simulink model "sdl_manual_transmission_TEST"  (R2015a)
settings: Solver=ode23t  StartTime=0.0  StopTime=30  MaxStep=0.1  RelTol=1e-3
PreLoadFcn:
  | L=0;
undefined symbols (not defined in the file): sigbuilder_block
libraries: fl_lib x47, nesl_utility x12, sdl_lib x8
Description:
  | Vehicle With Manual Transmission
  | 
  | The vehicle simulated in this demo has a four-speed manual transmission,
  | a schematic for which is available in the Gearbox subsystem. The key
  | elements of the transmission are four synchronizers, denoted by S_1 to
  | S_4. By engaging or disengaging these synchronizers and associated dog
  | clutches, the transmission provides four ratios 3.581, 2.022, 1.384, and 1,
  | respectively. The synchronizers are modeled using the Cone Clutch block.
  | The model also provides an alternative abstracted representation of the
  | gearbox more suitable for hardware-in-the-loop simulation. To select this,
  | right-click the Gearbox subsystem, and select Block Choice -> Gearbox
  | (Abstracted).
  | 
  | 
  | Copyright 2008-2014 The MathWorks, Inc.
settings Model: CovSFcnEnable=off  Creator=MathWorks  LastModifiedBy=psanghvi
settings SolverCC: MaxConsecutiveZCs=10  MaxConsecutiveMinStep=5
settings DataIOCC: SignalLoggingSaveFormat=ModelDataLogs
settings OptimizationCC: ExpressionDepthLimit=2147483647
settings DebuggingCC: UnderspecifiedInitializationDetection=Classic  MergeDetectMultiDrivingBlocksExec=none  MaxConsecutiveZCsMsg=none  IgnoredZcDiagnostic=none  FcnCallInpInsideContextMsg=UseLocalSettings  StateNameClashWarn=warning
settings GRTTargetCC: CombineOutputUpdateFcns=off  GRTInterface=on

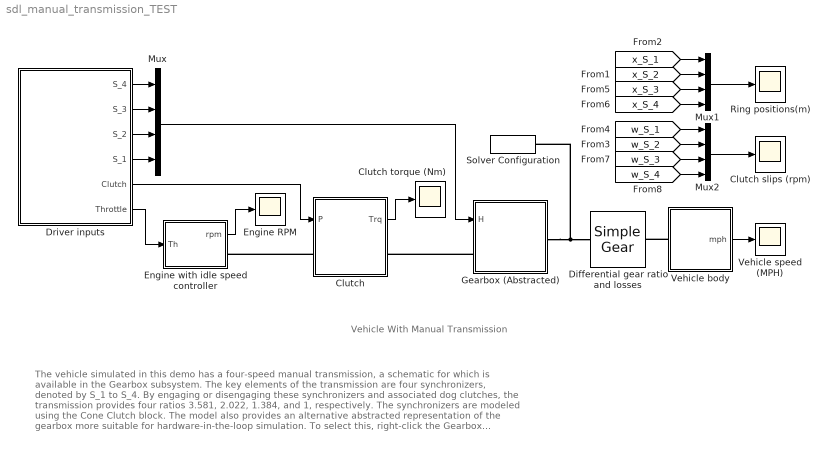
== system sdl_manual_transmission_TEST ==
  note: Vehicle With Manual Transmission
  note: The vehicle simulated in this demo has a four-speed manual transmission, a schematic for which is available in the Gearbox subsystem.
      | The key elements of the transmission are four synchronizers, denoted by S_1 to S_4. By engaging or disengaging these synchronizers and
      | associated dog clutches, the transmission provides four ratios 3.581, 2.022, 1.384, and 1, respectively. The synchronizers are modeled
      | using the Cone Clutch block. The model also provides an alternative abstracted representation of the gearbox more suitable for
      | hardware-in-the-loop simulation. To select this, right-click the Gearbox subsystem, and select Block Choice -> Gearbox (Abstracted).
  Clutch : Subsystem
  Clutch slips (rpm) : Scope
      settings: TimeRange=30  YMin=-2000  YMax=3000  SaveName=ScopeData8  MaxDataPoints=50000
  Clutch torque (Nm) : Scope
      settings: TimeRange=30  YMin=-50  YMax=300  SaveName=ScopeData4  MaxDataPoints=50000
  Differential gear ratio and losses : sdl_lib/Gears/Simple Gear  ratio=3.1  rotation_direction=1  friction_model=2  T_noload=0.1 N*m  T_nom=5 N*m  efficiency_nom=0.8  efficiency=0.86  mu_visc=[ L L ] N*m/(rad/s)  w_thr=0.01 rad/s  temperature_TLU=[ 280 300 320 ] K  load_TLU=[ 1 5 10 ] N*m  efficiency_TLU=[ 0.95 0.9 0.85 ]  efficiency_TLU2=[ 0.85 0.8 0.75; 0.95 0.9 0.85; 0.85 0.8 0.7 ]  thermal_mass=50 J/K  T_init=300 K
  Driver inputs : Subsystem  Tag=STV Subsys  LoadFcn=sigbuilder_block('load');  StartFcn=sigbuilder_block('start');  StopFcn=sigbuilder_block('stop');  ClipboardFcn=sigbuilder_block('clipboard');  mask(Sigbuilder block){}
      mask help: Sigbuilder GUI
      mask init:
      | if ~strcmp(get_param(bdroot(gcbh),'SimulationStatus'),'stopped') tuvar = sigbuilder_block('maskInit'); end
      settings: CopyFcn=sigbuilder_block('copy');  DeleteFcn=sigbuilder_block('delete');  ModelCloseFcn=sigbuilder_block('modelClose');  PreSaveFcn=sigbuilder_block('preSave');  PauseFcn=sigbuilder_block('pause')  ContinueFcn=sigbuilder_block('continue')  NameChangeFcn=sigbuilder_block('namechange');  OpenFcn=sigbuilder_block('open',[234.75 345 618.75 492 ]);  CloseFcn=sigbuilder_block('close');
      mask Display: plot(0,0,100,100,[10,10,40,40,10],[80,20,20,80,80],[40,10],[50,50], [40,27,10],[65,72,56],[40,25,25,10],[28,28,43,43]);
  Engine RPM : Scope
      settings: TimeRange=30  YMin=0  YMax=6000  SaveName=ScopeData6  MaxDataPoints=50000
  Engine with idle speed controller : Subsystem
  Gearbox (Abstracted) : Subsystem
  Mux : Mux
  Mux1 : Mux
  Mux2 : Mux
  Ring positions(m) : Scope
      settings: TimeRange=30  YMin=-0.005  YMax=0.015  SaveName=ScopeData7  MaxDataPoints=50000
  Solver Configuration : nesl_utility/Solver Configuration  PhysicalDomain=network_engine_domain  SubClassName=solver  LeftPortType=input  RightPortType=generic  Accelerate=off  Tones=[]  Harmonics=[]  SimulateNoise=off  Profile=off  UseLocalSampling=off  EnableSwitchedLinearOptims=on  FrequencyDomain=off  UseCCode=off  RelTol=0.001  AbsTol=1e-06  MinStep=1e-09  ToWorkspace=off  RevertToSquareIcSolve=off  NumHomotopyIterations=100  DoDC=off  ResidualTolerance=1e-9  UseLocalSolver=off  LocalSolverChoice=NE_BACKWARD_EULER_ADVANCER  LocalSolverSampleTime=.001  DoFixedCost=off  MaxNonlinIter=10  MaxModeIter=2  LinearAlgebra=Sparse  DelaysMemoryBudget=1024  AutomaticFiltering=on  FilteringTimeConstant=0.001
  Vehicle speed (MPH) : Scope
      settings: TimeRange=30  YMin=-20  YMax=80  SaveName=ScopeData5  MaxDataPoints=50000
  Vehicle body : Subsystem
  wires:
  Driver inputs/2(S_3) -> Mux/2
  Driver inputs/1(S_4) -> Mux/1
  Driver inputs/3(S_2) -> Mux/3
  Driver inputs/4(S_1) -> Mux/4
  Driver inputs/6(Throttle) -> Engine with idle speed controller/1(Th)
  Mux/1 -> Gearbox (Abstracted)/1(H)
  Driver inputs/5(Clutch) -> Clutch/1(P)
  Vehicle body/1(mph) -> Vehicle speed (MPH)/1
  Engine with idle speed controller/1(rpm) -> Engine RPM/1
  Clutch/1(Trq) -> Clutch torque (Nm)/1
  [x_S_1] -> Mux1/1
  [x_S_2] -> Mux1/2
  Mux1/1 -> Ring positions(m)/1
  Mux2/1 -> Clutch slips (rpm)/1
  [x_S_3] -> Mux1/3
  [x_S_4] -> Mux1/4
  [w_S_1] -> Mux2/1
  [w_S_2] -> Mux2/2
  [w_S_3] -> Mux2/3
  [w_S_4] -> Mux2/4
  connections:
  Clutch/LConn1 -- Engine with idle speed controller/RConn1
  Vehicle body/LConn1 -- Differential gear ratio and losses/RConn1
  Gearbox (Abstracted)/LConn1 -- Clutch/RConn1
  Gearbox (Abstracted)/RConn1 -- Differential gear ratio and losses/LConn1 -- Solver Configuration/RConn1

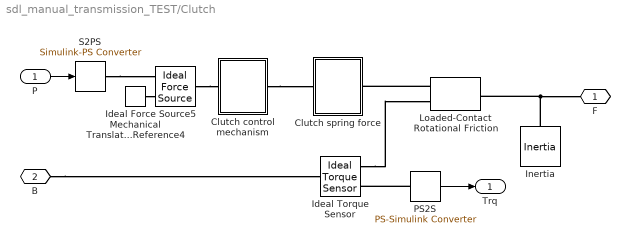
== system sdl_manual_transmission_TEST/Clutch ==
  P : Inport
  Clutch control mechanism : Subsystem
  Clutch spring force : Subsystem
  Ideal Torque Sensor : fl_lib/Mechanical/Mechanical Sensors/Ideal Torque Sensor
  Ideal Force Source5 : fl_lib/Mechanical/Mechanical Sources/Ideal Force Source
  Inertia : fl_lib/Mechanical/Rotational Elements/Inertia  inertia=0.005 kg*m^2  w_specify=on  w_priority=High  w=0 rad/s  t_specify=off  t_priority=High  t=0 N*m
  Loaded-Contact Rotational Friction : sdl_lib/Brakes & Detents/Rotational/Loaded-Contact Rotational Friction  geometry_model=1  r_eff=300 mm  d_o=150 mm  d_i=100 mm  friction_model=1  mu_coulomb=0.46  mu_w_vector=[ 0 0.1 0.2 0.3 0.4 0.5 1 2 5 10 100 1000 ] rad/s  mu_coulomb_vector=[ 0.29 0.28 0.26 0.22 0.21 0.2 0.2 0.19 0.19 0.19 0.19 0.19 ]  mu_interp_method=1  mu_extrap_method=1  mu_static=0.5  w_tol=0.001 rad/s  force_min=10 N  mu_visc=0 N*m/(rad/s)  initial_state_locked=0
  Mechanical Translational Reference4 : fl_lib/Mechanical/Translational Elements/Mechanical Translational Reference
  PS2S : nesl_utility/PS-Simulink Converter  PhysicalDomain=network_engine_domain  SubClassName=ps_output  LeftPortType=input  RightPortType=output  PseudoPeriodic=off  Frequencies=[]  Unit=1  AffineConversion=off
  S2PS : nesl_utility/Simulink-PS Converter  PhysicalDomain=network_engine_domain  SubClassName=ps_input  LeftPortType=input  RightPortType=output  PseudoPeriodic=off  Frequencies=[]  NoiseDistribution=none  NoiseParameters=[]  Unit=1  AffineConversion=off  InputFiltering=off  SimscapeFilterOrder=1  InputFilterTimeConstant=.001  UdotUserProvided=0
  F : PMIOPort  Port=1  Side=Right
  B : PMIOPort  Port=2  Side=Left
  Trq : Outport
  wires:
  P/1 -> S2PS/1
  PS2S/1 -> Trq/1
  connections:
  Mechanical Translational Reference4/LConn1 -- Ideal Force Source5/RConn2
  S2PS/RConn1 -- Ideal Force Source5/RConn1
  Ideal Force Source5/LConn1 -- Clutch control mechanism/LConn1
  Inertia/LConn1 -- Loaded-Contact Rotational Friction/RConn1 -- F/RConn1
  PS2S/LConn1 -- Ideal Torque Sensor/RConn2
  Clutch control mechanism/RConn1 -- Clutch spring force/LConn1
  Loaded-Contact Rotational Friction/LConn1 -- Clutch spring force/RConn1
  Ideal Torque Sensor/RConn1 -- Loaded-Contact Rotational Friction/LConn2
  B/RConn1 -- Ideal Torque Sensor/LConn1

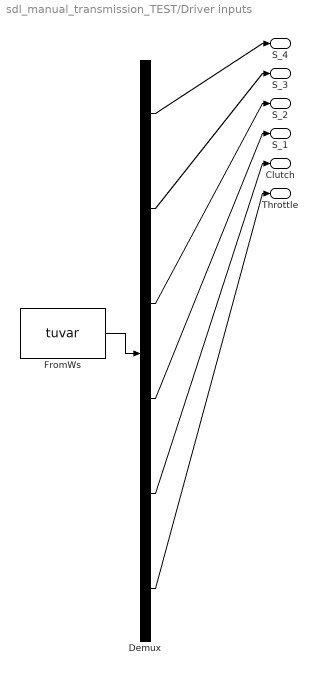
== system sdl_manual_transmission_TEST/Driver inputs ==
  Demux : Demux  Tag=STV Demux  Outputs=6
  FromWs : FromWorkspace  Tag=STV FromWs  VariableName=tuvar  SampleTime=0
      SigBuilderData=|
      | common.afterFinalStr = 'Extrapolate'
      | common.sampleTime = 0
      | dataSet.timeRange = [0 30]
      | dataSet.name = 'Group 1'
      | sbobj.Groups.Name = 'Group 1'
      | sbobj.Groups.Signals(1).Name = 'S_4'
      | sbobj.Groups.Signals(1).XData = [0 23.3 23.5 24 24.3 30]
      | sbobj.Groups.Signals(1).YData = [0 0 250 250 0 0]
      | sbobj.Groups.Signals(2).Name = 'S_3'
      | sbobj.Groups.Signals(2).XData = [0 16.1 16.3 16.9 17.2 22.8 23 23.6 23.7 30]
      | sbobj.Groups.Signals(2).YData = [0 0 250 250 0 0 -250 -250 0 0]
      | sbobj.Groups.Signals(3).Name = 'S_2'
      | sbobj.Groups.Signals(3).XData = [0 8.8 9 9.5 9.75 15.8 16.05 16.6 16.8 30]
      | sbobj.Groups.Signals(3).YData = [0 0 250 250 0 0 -250 -250 0 0]
      | sbobj.Groups.Signals(4).Name = 'S_1'
      | sbobj.Groups.Signals(4).XData = [0 1.7 1.85 3.15 3.35 8.35 8.5 9.3 9.4 30]
      | sbobj.Groups.Signals(4).YData = [0 0 250 250 0 0 -250 -250 0 0]
      | sbobj.Groups.Signals(5).Name = 'Clutch'
      | sbobj.Groups.Signals(5).XData = [0 0.95 1.45 3.5 4 8.15 8.35 10 10.4 15.4 15.8 17.2 17.7 22.5 22.8 24.3 24.6 30]
      | sbobj.Groups.Signals(5).YData = [0 0 120 120 -0.05 0 120 120 0 0 120 120 0 0 120 120 0 0]
      | sbobj.Groups.Signals(6).Name = 'Throttle'
      | sbobj.Groups.Signals(6).XData = [0 3.2 4 7.45 7.6 10.25 10.4 15 15.2 17.6 17.8 22.35 22.6 24.6 24.8 30]
      | sbobj.Groups.Signals(6).YData = [0 0 0.95 0.95 0 0 0.96 0.943121387283 0 0 1 1 0 0 1 1]
      | sbobj.Groups.TimeRange = [0 30]
  S_4 : Outport  Tag=STV Outport
  S_3 : Outport  Tag=STV Outport  Port=2
  S_2 : Outport  Tag=STV Outport  Port=3
  S_1 : Outport  Tag=STV Outport  Port=4
  Clutch : Outport  Tag=STV Outport  Port=5
  Throttle : Outport  Tag=STV Outport  Port=6
  wires:
  Demux/6 -> Throttle/1
  Demux/5 -> Clutch/1
  Demux/4 -> S_1/1
  Demux/3 -> S_2/1
  Demux/2 -> S_3/1
  Demux/1 -> S_4/1
  FromWs/1 -> Demux/1

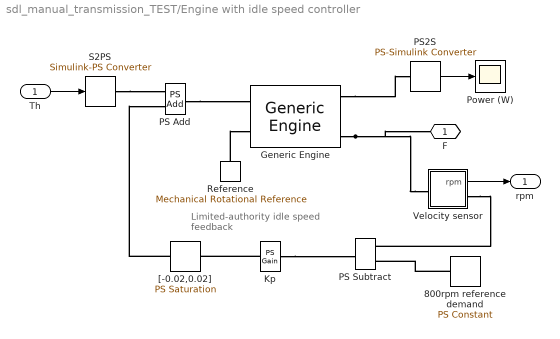
== system sdl_manual_transmission_TEST/Engine with idle speed controller ==
  note: Limited-authority
      | idle speed feedback
  Th : Inport
  800rpm reference demand : fl_lib/Physical Signals/Sources/PS Constant  constant=800*2*pi/60
  Generic Engine : sdl_lib/Engines/Generic Engine  model_parameterization=1  engine_type=1  P_max=100e3 W  w_P_max=4.5e+3 rpm  w_max=6e+3 rpm  w_min=200 rpm  w_tab=[ 500 1000 2e+3 3e+3 4e+3 5e+3 6e+3 7e+3 ] rpm  trq_tab=[ 380 380 380 380 350 280 200 80 ] N*m  pwr_tab=[ 2e+4 4e+4 7.8e+4 1.2e+5 1.45e+5 1.48e+5 1.25e+5 6e+4 ] W  interp_method=1  model_inertia=1  inertia=0.08 kg*m^2  initial_velocity=800 rpm  model_time_constant=1  time_constant=0.2 s  T0=0  w_thr=20 rpm  idle_speed=0  idle_speed_reference=1000 rpm  tau_controller=1 s  idle_w_thr=1 rpm  fc_model=1  fc_per_rev=25 mg/rev  displaced_volume=400 cm^3  rev_per_cycle=2  fc_w_tab=[ 1000 2e+3 3e+3 4e+3 5e+3 6e+3 ] rpm  fc_trq_tab=[ 0 80 160 200 240 320 360 400 ] N*m  fc_tab=[ 0.5 0.9 1.4 1.6 1.9 2.7 3.4 4.4; 1 1.7 2.7 3.1 3.6 5 6 7.4; 1.4 2.7 4 4.8 5.6 7.5 8.5 10.5; 2 3.6 5.8 6.7 8 10.4 11.7 13.3; 2.5 4.8 7.9 9.4 10.8 14 16.2 18.6; 3.1 6 10.3 11.9 13.8 18.4 22 26.5 ] g/s  bmep_tab=[ 0 250 500 625 750 1000 1.15e+3 1.25e+3 ] kPa  bsfc_tab=[ 410 380 300 280 270 290 320 380; 410 370 290 270 260 270 285 320; 415 380 290 275 265 270 270 300; 420 390 310 290 285 280 280 285; 430 410 340 320 310 300 310 320; 450 430 370 340 330 330 350 380 ] g/hr/kW  fc_interp_method=1
  Kp : fl_lib/Physical Signals/Functions/PS Gain  gain=0.005
  PS Add : fl_lib/Physical Signals/Functions/PS Add
  PS Subtract : fl_lib/Physical Signals/Functions/PS Subtract
  PS2S : nesl_utility/PS-Simulink Converter  PhysicalDomain=network_engine_domain  SubClassName=ps_output  LeftPortType=input  RightPortType=output  PseudoPeriodic=off  Frequencies=[]  Unit=1  AffineConversion=off
  Power (W) : Scope
      settings: TimeRange=15  YMin=-50000  YMax=150000  SaveName=ScopeData2
  Reference : fl_lib/Mechanical/Rotational Elements/Mechanical Rotational Reference
  S2PS : nesl_utility/Simulink-PS Converter  PhysicalDomain=network_engine_domain  SubClassName=ps_input  LeftPortType=input  RightPortType=output  PseudoPeriodic=off  Frequencies=[]  NoiseDistribution=none  NoiseParameters=[]  Unit=1  AffineConversion=off  InputFiltering=off  SimscapeFilterOrder=1  InputFilterTimeConstant=.001  UdotUserProvided=0
  Velocity sensor : Subsystem
  "[-0.02,0.02]" : fl_lib/Physical Signals/Nonlinear Operators/PS Saturation  upper_limit=0.02  lower_limit=-0.02
  F : PMIOPort  Port=1  Side=Right
  rpm : Outport
  wires:
  Velocity sensor/1(rpm) -> rpm/1
  PS2S/1 -> Power (W)/1
  Th/1 -> S2PS/1
  connections:
  Generic Engine/RConn1 -- PS2S/LConn1
  Reference/LConn1 -- Generic Engine/LConn2
  PS Add/RConn1 -- Generic Engine/LConn1
  S2PS/RConn1 -- PS Add/LConn1
  Velocity sensor/RConn1 -- PS Subtract/LConn2
  800rpm reference demand/RConn1 -- PS Subtract/LConn1
  Kp/LConn1 -- PS Subtract/RConn1
  "[-0.02,0.02]"/RConn1 -- PS Add/LConn2
  Kp/RConn1 -- "[-0.02,0.02]"/LConn1
  Velocity sensor/LConn1 -- Generic Engine/RConn3 -- F/RConn1

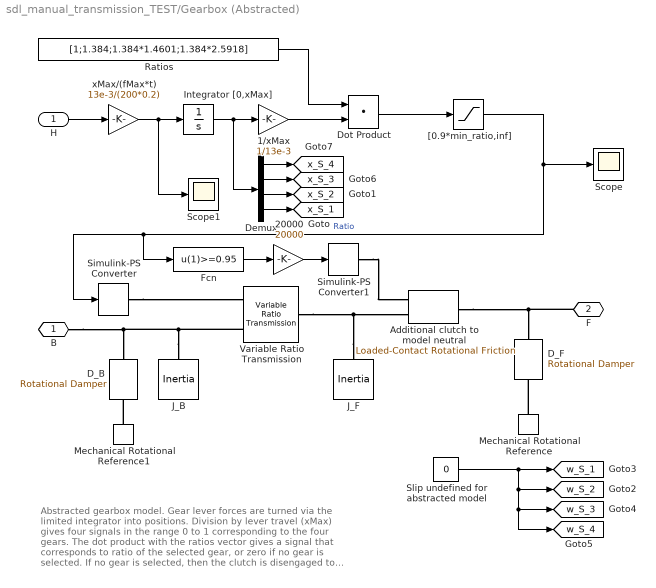
== system sdl_manual_transmission_TEST/Gearbox (Abstracted) ==
  note: Abstracted gearbox model. Gear lever forces are turned
      | via the limited integrator into positions. Division
      | by lever travel (xMax) gives four signals in the range
      | 0 to 1 corresponding to the four gears. The dot
      | product with the ratios vector gives a signal that
      | corresponds to ratio of the selected gear, or zero if
      | no gear is selected. If no gear is selected, then the
      | clutch is disengaged to represent neutral.
  H : Inport
  1/xMax : Gain  Gain=1/13e-3  SaturateOnIntegerOverflow=on  OutDataTypeStr=Inherit: Same as input  ParamDataTypeStr=Inherit: Same as input
  20000 : Gain  Gain=20000  SaturateOnIntegerOverflow=on  OutDataTypeStr=Inherit: Same as input  ParamDataTypeStr=Inherit: Same as input
  Additional clutch to model neutral : sdl_lib/Brakes & Detents/Rotational/Loaded-Contact Rotational Friction  geometry_model=1  r_eff=300 mm  d_o=150 mm  d_i=100 mm  friction_model=1  mu_coulomb=0.46  mu_w_vector=[ 0 0.1 0.2 0.3 0.4 0.5 1 2 5 10 100 1000 ] rad/s  mu_coulomb_vector=[ 0.29 0.28 0.26 0.22 0.21 0.2 0.2 0.19 0.19 0.19 0.19 0.19 ]  mu_interp_method=1  mu_extrap_method=1  mu_static=0.5  w_tol=0.001 rad/s  force_min=100 N  mu_visc=0 N*m/(rad/s)  initial_state_locked=0
  D_B : fl_lib/Mechanical/Rotational Elements/Rotational Damper  D=0.01 N*m/(rad/s)  w_specify=off  w_priority=High  w=0 rad/s  t_specify=off  t_priority=High  t=0 N*m
  D_F : fl_lib/Mechanical/Rotational Elements/Rotational Damper  D=0.01 N*m/(rad/s)  w_specify=off  w_priority=High  w=0 rad/s  t_specify=off  t_priority=High  t=0 N*m
  Demux : Demux
  Dot Product : DotProduct  OutDataTypeStr=Inherit: Inherit via internal rule
  Fcn : Fcn  Expr=u(1)>=0.95
  Integrator [0,xMax] : Integrator  LimitOutput=on  UpperSaturationLimit=13e-3  LowerSaturationLimit=0
  J_B : fl_lib/Mechanical/Rotational Elements/Inertia  inertia=0.026 kg*m^2  w_specify=on  w_priority=High  w=0 rad/s  t_specify=off  t_priority=High  t=0 N*m
  J_F : fl_lib/Mechanical/Rotational Elements/Inertia  inertia=0.034 kg*m^2  w_specify=on  w_priority=High  w=0 rad/s  t_specify=off  t_priority=High  t=0 N*m
  Mechanical Rotational Reference : fl_lib/Mechanical/Rotational Elements/Mechanical Rotational Reference
  Mechanical Rotational Reference1 : fl_lib/Mechanical/Rotational Elements/Mechanical Rotational Reference
  Ratios : Constant  Value=[1;1.384;1.384*1.4601;1.384*2.5918]  VectorParams1D=off
  Scope : Scope
  Scope1 : Scope
      settings: SaveName=ScopeData9
  Simulink-PS Converter : nesl_utility/Simulink-PS Converter  PhysicalDomain=network_engine_domain  SubClassName=ps_input  LeftPortType=input  RightPortType=output  PseudoPeriodic=off  Frequencies=[]  NoiseDistribution=none  NoiseParameters=[]  Unit=1  AffineConversion=off  InputFiltering=off  SimscapeFilterOrder=1  InputFilterTimeConstant=.001  UdotUserProvided=0
  Simulink-PS Converter1 : nesl_utility/Simulink-PS Converter  PhysicalDomain=network_engine_domain  SubClassName=ps_input  LeftPortType=input  RightPortType=output  PseudoPeriodic=off  Frequencies=[]  NoiseDistribution=none  NoiseParameters=[]  Unit=1  AffineConversion=off  InputFiltering=off  SimscapeFilterOrder=1  InputFilterTimeConstant=.001  UdotUserProvided=0
  Slip undefined for abstracted model : Constant  Value=0
  Variable Ratio Transmission : sdl_lib/Couplings & Drives/Variable Ratio Transmission  rotation_direction=1  kp=1e+5 N*m/rad  kv=10 N*m/(rad/s)  initial_torque=0 N*m  losses_model=1  efficiency=0.85  mu_visc=[ 0 0 ] N*m/(rad/s)  w_thr=0.01 rad/s
  "[0.9*min_ratio,inf]" : Saturate  UpperLimit=inf  LowerLimit=0.9
  xMax/(fMax*t) : Gain  Gain=13e-3/(200*0.2)  SaturateOnIntegerOverflow=on  OutDataTypeStr=Inherit: Same as input  ParamDataTypeStr=Inherit: Same as input
  B : PMIOPort  Port=1  Side=Left
  F : PMIOPort  Port=2  Side=Right
  tag scope: w_S_1=global, w_S_2=global, w_S_3=global, w_S_4=global, x_S_1=global, x_S_2=global, x_S_3=global, x_S_4=global
  wires:
  Dot Product/1 -> "[0.9*min_ratio,inf]"/1
  Ratios/1 -> Dot Product/1
  1/xMax/1 -> Dot Product/2
  Integrator [0,xMax]/1 -> 1/xMax/1, Demux/1
  xMax/(fMax*t)/1 -> Integrator [0,xMax]/1, Scope1/1
  H/1 -> xMax/(fMax*t)/1
  Demux/4 -> [x_S_1]
  Demux/3 -> [x_S_2]
  Demux/1 -> [x_S_4]
  Demux/2 -> [x_S_3]
  "[0.9*min_ratio,inf]"/1 -> Simulink-PS Converter/1, Fcn/1, Scope/1  "Ratio"
  Fcn/1 -> 20000/1
  20000/1 -> Simulink-PS Converter1/1
  Slip undefined for abstracted model/1 -> [w_S_4], [w_S_3], [w_S_2], [w_S_1]
  connections:
  F/RConn1 -- D_F/LConn1 -- Additional clutch to model neutral/RConn1
  Mechanical Rotational Reference1/LConn1 -- D_B/RConn1
  Mechanical Rotational Reference/LConn1 -- D_F/RConn1
  J_B/LConn1 -- D_B/LConn1 -- B/RConn1 -- Variable Ratio Transmission/LConn2
  Simulink-PS Converter/RConn1 -- Variable Ratio Transmission/LConn1
  J_F/LConn1 -- Additional clutch to model neutral/LConn2 -- Variable Ratio Transmission/RConn1
  Simulink-PS Converter1/RConn1 -- Additional clutch to model neutral/LConn1

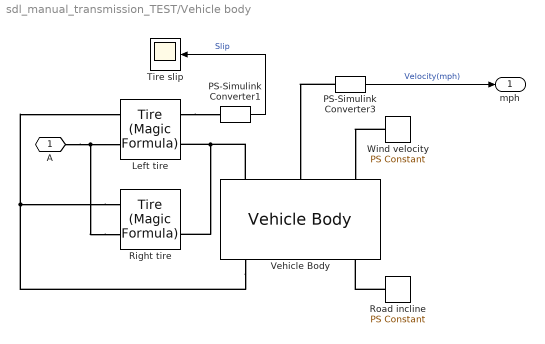
== system sdl_manual_transmission_TEST/Vehicle body ==
  Left tire : sdl_lib/Tires & Vehicles/Tire (Magic Formula)  parameterization=3  F_z1=3000 N  F_x1=3500 N  kappa1=10  B_m=10  C_m=1.9  D_m=1  E_m=0.97  fz0=4e+3 N  p_Cx=1.685  p_Dx=[ 1.21 -0.037 ]  p_Ex=[ 0.344 0.095 -0.02 0 ]  p_Kx=[ 21.51 -0.163 0.245 ]  p_Hx=[ -0.002 0.002 ]  p_Vx=[ 0 0 ]  v_tr_thr=0.1 m/s  r_e=0.4 m  model_compliance=0  stiffness=1e+6 N/m  damping=1000 N/(m/s)  model_inertia=1  inertia=0.8 kg*m^2  initial_velocity=0 rpm  model_resistance=0  resistance_model=1  coeff=0.015  p_tire=250e3 Pa  alpha=-0.003  beta=0.97  coeff_a=84e-4  coeff_b=6.2e-4 s/m  coeff_c=1.6e-4 s^2/m^2  v_thr=1e-3 m/s
  PS-Simulink Converter1 : nesl_utility/PS-Simulink Converter  PhysicalDomain=network_engine_domain  SubClassName=ps_output  LeftPortType=input  RightPortType=output  PseudoPeriodic=off  Frequencies=[]  Unit=1  AffineConversion=off
  PS-Simulink Converter3 : nesl_utility/PS-Simulink Converter  PhysicalDomain=network_engine_domain  SubClassName=ps_output  LeftPortType=input  RightPortType=output  PseudoPeriodic=off  Frequencies=[]  Unit=mph  AffineConversion=off
  Right tire : sdl_lib/Tires & Vehicles/Tire (Magic Formula)  parameterization=3  F_z1=3000 N  F_x1=3500 N  kappa1=10  B_m=10  C_m=1.9  D_m=1  E_m=0.97  fz0=4e+3 N  p_Cx=1.685  p_Dx=[ 1.21 -0.037 ]  p_Ex=[ 0.344 0.095 -0.02 0 ]  p_Kx=[ 21.51 -0.163 0.245 ]  p_Hx=[ -0.002 0.002 ]  p_Vx=[ 0 0 ]  v_tr_thr=0.1 m/s  r_e=0.4 m  model_compliance=0  stiffness=1e+6 N/m  damping=1000 N/(m/s)  model_inertia=1  inertia=0.8 kg*m^2  initial_velocity=0 rpm  model_resistance=0  resistance_model=1  coeff=0.015  p_tire=250e3 Pa  alpha=-0.003  beta=0.97  coeff_a=84e-4  coeff_b=6.2e-4 s/m  coeff_c=1.6e-4 s^2/m^2  v_thr=1e-3 m/s
  Road incline : fl_lib/Physical Signals/Sources/PS Constant  constant=0
  Tire slip : Scope
      settings: YMin=0  YMax=0.1  SaveName=ScopeData3  MaxDataPoints=500000  SampleTime=0.1
  Vehicle Body : sdl_lib/Tires & Vehicles/Vehicle Body  mass=1200 kg  n_w=2  x_f=1.4 m  x_r=1.6 m  y_c=0.5 m  area=3 m^2  Cd=0.4  v0=0 m/s  g=9.81 m/s^2  rho=1.18 kg/m^3
  Wind velocity : fl_lib/Physical Signals/Sources/PS Constant  constant=5
  A : PMIOPort  Port=1  Side=Left
  mph : Outport
  wires:
  PS-Simulink Converter3/1 -> mph/1  "Velocity(mph)"
  PS-Simulink Converter1/1 -> Tire slip/1  "Slip"
  connections:
  Right tire/RConn2 -- Left tire/RConn2 -- Vehicle Body/LConn1
  Right tire/LConn1 -- Left tire/LConn1 -- Vehicle Body/RConn1
  Right tire/LConn2 -- Left tire/LConn2 -- A/RConn1
  PS-Simulink Converter3/LConn1 -- Vehicle Body/LConn2
  Wind velocity/RConn1 -- Vehicle Body/LConn3
  Road incline/RConn1 -- Vehicle Body/RConn3
  Left tire/RConn1 -- PS-Simulink Converter1/LConn1

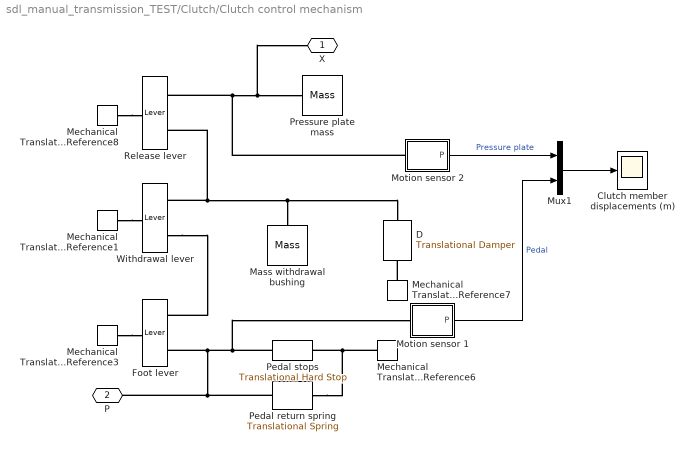
== system sdl_manual_transmission_TEST/Clutch/Clutch control mechanism ==
  Clutch member displacements (m) : Scope
      settings: TimeRange=15  YMin=-0.05  YMax=0.2  MaxDataPoints=50000
  D : fl_lib/Mechanical/Translational Elements/Translational Damper  D=100 N/(m/s)  v_specify=off  v_priority=High  v=0 m/s  f_specify=off  f_priority=High  f=0 N
  Foot lever : fl_lib/Mechanical/Mechanisms/Lever  arm_AC=76 mm  arm_BC=148 mm  f_A_specify=off  f_A_priority=High  f_A=0 N  f_B_specify=off  f_B_priority=High  f_B=0 N  f_C_specify=off  f_C_priority=High  f_C=0 N
  Mass withdrawal bushing : fl_lib/Mechanical/Translational Elements/Mass  mass=0.6 kg  v_specify=on  v_priority=High  v=0 m/s  f_specify=off  f_priority=High  f=0 N
  Mechanical Translational Reference{1,3,6..8} (5 alike) : fl_lib/Mechanical/Translational Elements/Mechanical Translational Reference
  Motion sensor 1 : Subsystem
  Motion sensor 2 : Subsystem
  Mux1 : Mux  Inputs=2
  Pedal return spring : fl_lib/Mechanical/Translational Elements/Translational Spring  spr_rate=120 N/m  v_specify=off  v_priority=High  v=0 m/s  f_specify=off  f_priority=High  f=0 N  x_specify=on  x_priority=High  x=1.5 cm
  Pedal stops : fl_lib/Mechanical/Translational Elements/Translational Hard Stop  upper_bnd=168 mm  lower_bnd=0 mm  stiff_up=1e6 N/m  stiff_low=1e6 N/m  D_up=150 N/(m/s)  D_low=150 N/(m/s)  v_specify=off  v_priority=High  v=0 m/s  f_specify=off  f_priority=High  f=0 N  x_specify=on  x_priority=High  x=0 m
  Pressure plate mass : fl_lib/Mechanical/Translational Elements/Mass  mass=4.2 kg  v_specify=on  v_priority=High  v=0 m/s  f_specify=off  f_priority=High  f=0 N
  Release lever : fl_lib/Mechanical/Mechanisms/Lever  arm_AC=7.2 mm  arm_BC=38 mm  f_A_specify=off  f_A_priority=High  f_A=0 N  f_B_specify=off  f_B_priority=High  f_B=0 N  f_C_specify=off  f_C_priority=High  f_C=0 N
  Withdrawal lever : fl_lib/Mechanical/Mechanisms/Lever  arm_AC=42 mm  arm_BC=128 mm  f_A_specify=off  f_A_priority=High  f_A=0 N  f_B_specify=off  f_B_priority=High  f_B=0 N  f_C_specify=off  f_C_priority=High  f_C=0 N
  X : PMIOPort  Port=1  Side=Right
  P : PMIOPort  Port=2  Side=Left
  wires:
  Motion sensor 2/1(P) -> Mux1/1  "Pressure plate"
  Motion sensor 1/1(P) -> Mux1/2  "Pedal"
  Mux1/1 -> Clutch member displacements (m)/1
  connections:
  Mechanical Translational Reference3/LConn1 -- Foot lever/RConn1
  Mechanical Translational Reference6/LConn1 -- Pedal stops/RConn1 -- Pedal return spring/RConn1
  Mechanical Translational Reference7/LConn1 -- D/RConn1
  Mechanical Translational Reference8/LConn1 -- Release lever/RConn1
  Withdrawal lever/LConn2 -- Foot lever/LConn1
  Mechanical Translational Reference1/LConn1 -- Withdrawal lever/RConn1
  Withdrawal lever/LConn1 -- Release lever/LConn2 -- Mass withdrawal bushing/LConn1 -- D/LConn1
  Motion sensor 2/LConn1 -- Release lever/LConn1 -- X/RConn1 -- Pressure plate mass/LConn1
  Pedal stops/LConn1 -- Foot lever/LConn2 -- Pedal return spring/LConn1 -- P/RConn1 -- Motion sensor 1/LConn1

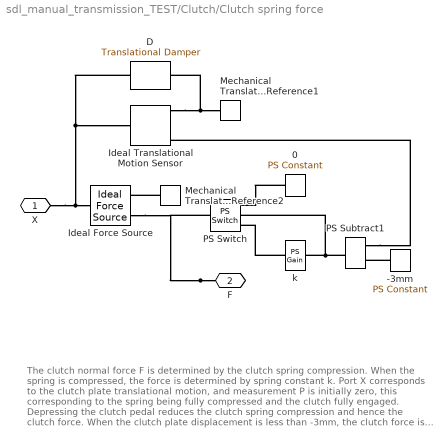
== system sdl_manual_transmission_TEST/Clutch/Clutch spring force ==
  note: The clutch normal force F is determined by the clutch spring compression.
      | When the spring is compressed, the force is determined by spring constant
      | k. Port X corresponds to the clutch plate translational motion, and
      | measurement P is initially zero, this corresponding to the spring being
      | fully compressed and the clutch fully engaged. Depressing the clutch pedal
      | reduces the clutch spring compression and hence the clutch force. When the
      | clutch plate displacement is less than -3mm, the clutch force is zero, and
      | hence it is fully disengaged.
  -3mm : fl_lib/Physical Signals/Sources/PS Constant  constant=-3e-3
  0 : fl_lib/Physical Signals/Sources/PS Constant  constant=0
  D : fl_lib/Mechanical/Translational Elements/Translational Damper  D=100 N/(m/s)  v_specify=off  v_priority=High  v=0 m/s  f_specify=off  f_priority=High  f=0 N
  Ideal Force Source : fl_lib/Mechanical/Mechanical Sources/Ideal Force Source
  Ideal Translational Motion Sensor : fl_lib/Mechanical/Mechanical Sensors/Ideal Translational Motion Sensor  offset=0 m
  Mechanical Translational Reference1 : fl_lib/Mechanical/Translational Elements/Mechanical Translational Reference
  Mechanical Translational Reference2 : fl_lib/Mechanical/Translational Elements/Mechanical Translational Reference
  PS Subtract1 : fl_lib/Physical Signals/Functions/PS Subtract
  PS Switch : fl_lib/Physical Signals/Nonlinear Operators/PS Switch  Threshold=0
  k : fl_lib/Physical Signals/Functions/PS Gain  gain=2000/3e-3
  X : PMIOPort  Port=1  Side=Left
  F : PMIOPort  Port=2  Side=Right
  connections:
  Ideal Translational Motion Sensor/RConn1 -- Mechanical Translational Reference1/LConn1 -- D/RConn1
  PS Subtract1/LConn1 -- Ideal Translational Motion Sensor/RConn3
  D/LConn1 -- X/RConn1 -- Ideal Force Source/LConn1 -- Ideal Translational Motion Sensor/LConn1
  F/RConn1 -- Ideal Force Source/RConn1 -- PS Switch/RConn1
  Mechanical Translational Reference2/LConn1 -- Ideal Force Source/RConn2
  PS Subtract1/RConn1 -- k/LConn1 -- PS Switch/LConn2
  k/RConn1 -- PS Switch/LConn1
  0/RConn1 -- PS Switch/LConn3
  -3mm/RConn1 -- PS Subtract1/LConn2

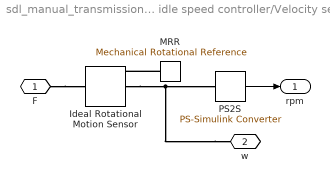
== system sdl_manual_transmission_TEST/Engine with idle speed controller/Velocity sensor ==
  Ideal Rotational Motion Sensor : fl_lib/Mechanical/Mechanical Sensors/Ideal Rotational Motion Sensor  offset=0 rad
  MRR : fl_lib/Mechanical/Rotational Elements/Mechanical Rotational Reference
  PS2S : nesl_utility/PS-Simulink Converter  PhysicalDomain=network_engine_domain  SubClassName=ps_output  LeftPortType=input  RightPortType=output  PseudoPeriodic=off  Frequencies=[]  Unit=rpm  AffineConversion=off
  F : PMIOPort  Port=1  Side=Left
  w : PMIOPort  Port=2  Side=Right
  rpm : Outport
  wires:
  PS2S/1 -> rpm/1
  connections:
  F/RConn1 -- Ideal Rotational Motion Sensor/LConn1
  w/RConn1 -- Ideal Rotational Motion Sensor/RConn2 -- PS2S/LConn1
  MRR/LConn1 -- Ideal Rotational Motion Sensor/RConn1

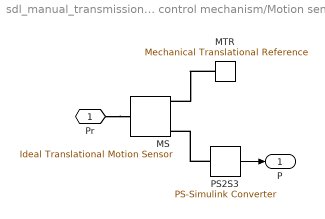
== system sdl_manual_transmission_TEST/Clutch/Clutch control mechanism/Motion sensor 1 ==
  MS : fl_lib/Mechanical/Mechanical Sensors/Ideal Translational Motion Sensor  offset=0 m
  MTR : fl_lib/Mechanical/Translational Elements/Mechanical Translational Reference
  PS2S3 : nesl_utility/PS-Simulink Converter  PhysicalDomain=network_engine_domain  SubClassName=ps_output  LeftPortType=input  RightPortType=output  PseudoPeriodic=off  Frequencies=[]  Unit=1  AffineConversion=off
  Pr : PMIOPort  Port=1  Side=Left
  P : Outport
  wires:
  PS2S3/1 -> P/1
  connections:
  MTR/LConn1 -- MS/RConn1
  PS2S3/LConn1 -- MS/RConn3
  Pr/RConn1 -- MS/LConn1

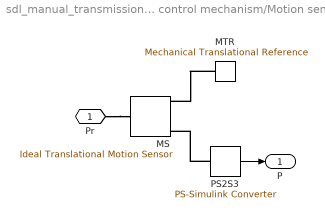
== system sdl_manual_transmission_TEST/Clutch/Clutch control mechanism/Motion sensor 2 ==
  MS : fl_lib/Mechanical/Mechanical Sensors/Ideal Translational Motion Sensor  offset=0 m
  MTR : fl_lib/Mechanical/Translational Elements/Mechanical Translational Reference
  PS2S3 : nesl_utility/PS-Simulink Converter  PhysicalDomain=network_engine_domain  SubClassName=ps_output  LeftPortType=input  RightPortType=output  PseudoPeriodic=off  Frequencies=[]  Unit=1  AffineConversion=off
  Pr : PMIOPort  Port=1  Side=Left
  P : Outport
  wires:
  PS2S3/1 -> P/1
  connections:
  Pr/RConn1 -- MS/LConn1
  PS2S3/LConn1 -- MS/RConn3
  MTR/LConn1 -- MS/RConn1
